simulink library "avalon_mm_alteradspbuilder2"  (Simulink 7.6)
settings: Solver=ode45  StartTime=0.0  StopTime=10.0  RelTol=1e-3
InitFcn:
  | %% DSPBuilder Start
  | alt_dspbuilder_update_model(bdroot)
  | %% DSPBuilder End
libraries: allblocks_alteradspbuilder2 x17
settings Model: Creator=swbuild  LastModifiedBy=swbuild

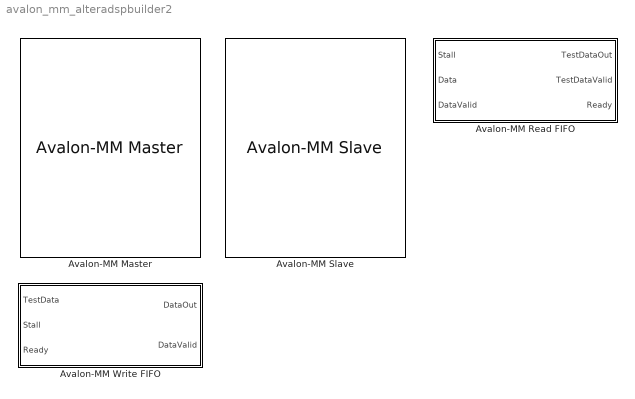
== system avalon_mm_alteradspbuilder2 ==
  Avalon-MM Master : allblocks_alteradspbuilder2/Avalon-MM Master  SystemSampleTime=-1  iofile=D:\avalon%5Fmm%5Falteradspbuilder2_Avalon-MM+Master_waitrequest.salt,D:\avalon%5Fmm%5Falteradspbuilder2_Avalon-MM+Master_address.capture,D:\avalon%5Fmm%5Falteradspbuilder2_Avalon-MM+Master_read.capture,D:\avalon%5Fmm%5Falteradspbuilder2_Avalon-MM+Master_readdata.salt,  SpecifyClock=off  addrWidth=2  addrType=Read  BusType=Signed Integer  bwl=8  bwr=0  byteEnable=off  flowCtrl=off  pipeline=off  flush=off  burst=off  maxBurst=4  irq=off  irq_mode=Prioritized  externalType=Inferred  PORTTYPE=Input
  Avalon-MM Read FIFO : Subsystem  mask(Avalon-MM Read FIFO AlteraBlockSet){sgn=Signed Integer, bwl=8, bwr=3, depth=11, burst=0}
      mask prompts: sgn "Data Type"; bwl "[number of bits].[]"; bwr "[].[number of bits]"; depth "FIFO Depth"; burst "Max Burst"
      mask help:
      | Avalon-MM Read FIFO
      |
      | Implements a FIFO with Avalon-MM connectivity. Accessed by other Avalon-MM peripherals to obtain datawhen connected in SOPC Builder.
      |
      | Inputs:
      | Stall - Connect to Simulink blocks.
      | 	Used to simulate stall conditions of the Avalon-MM bus.
      | Data - Connect to DSP Builder blocks.
      | 	Used to collect outgoing data from the user design.
      | DataValid - Connect to DSP Builder blocks.
      | 	Should be asserted whenever the signal on the Data port corresponds to real data.
      |
      | Outputs:
      | TestDataOut - Connect to Simulink blocks.
      | 	Corresponds to the data received over the Avalon-MM bus.
      | TestDataValid - Connect to Simulink blocks.
      | 	Asserted whenever TestDataOut corresponds to real data.
      | Ready	- Connect to DSP Builder blocks.
      | 	Used to indicate that the block is ready to receive data.
      mask init:
      | alt_dspbuilder_internal_AvalonFIFO_Init(gcb,1,1, bwl,bwr,depth,burst);
      settings: CopyFcn=set_param(gcbh,'LinkStatus','none');
      mask Help: helpview(fullfile(alt_dspbuilder_get_quartus_rootdir, 'dsp_builder', 'docs', 'AvalonReadFIFO.html'))
      mask StyleString: popup(Signed Integer|Signed Fractional|Unsigned Integer),edit,edit,edit,edit
      mask CallbackString: alt_dspbuilder_internal_AvalonFIFO_Init(gcb,1,0);||||
  Avalon-MM Slave : allblocks_alteradspbuilder2/Avalon-MM Slave  SystemSampleTime=-1  iofile=d:\SJ\nightly\13.1\162\w32\acds\quartus\dsp_builder\bin\mdllibrary\tb_avalon_mm_alteradspbuilder2\avalon%5Fmm%5Falteradspbuilder2_Avalon-MM+Slave_address.salt,d:\SJ\nightly\13.1\162\w32\acds\quartus\dsp_builder\bin\mdllibrary\tb_avalon_mm_alteradspbuilder2\avalon%5Fmm%5Falteradspbuilder2_Avalon-MM+Slave_write.salt,d:\SJ\nightly\13.1\162\w32\acds\quartus\dsp_builder\bin\mdllibrary\tb_avalon_mm_alteradspbuilder2\avalon%5Fmm%5Falteradspbuilder2_Avalon-MM+Slave_writedata.salt,d:\SJ\nightly\13.1\162\w32\acds\quartus\dsp_builder\bin\mdllibrary\tb_avalon_mm_alteradspbuilder2\avalon%5Fmm%5Falteradspbuilder2_Avalon-MM+Slave_byteenable.salt,  SpecifyClock=off  addrWidth=2  addrAlignment=Dynamic  addrType=Write  BusType=Unsigned Integer  bwl=16  bwr=0  byteEnable=on  flowCtrl=off  pipeline=off  waitStateFormat=Fixed  readWaitStateCycles=0  writeWaitStateCycles=0  readLatencyFormat=Fixed  readLatencyCycles=0  burst=off  maxBurst=4  irq=off  receiveBeginTransfer=off  useChipSelect=off  externalType=Inferred  PORTTYPE=Output
  Avalon-MM Write FIFO : Subsystem  mask(Avalon-MM Write FIFO AlteraBlockSet){sgn=Unsigned Integer, bwl=8, bwr=0, depth=16, burst=8}
      mask prompts: sgn "Data Type"; bwl "[number of bits].[]"; bwr "[].[number of bits]"; depth "FIFO Depth"; burst "Maximum Burst Size"
      mask help:
      | Avalon-MM Write FIFO
      |
      | Implements a FIFO with Avalon-MM connectivity. Used to receive data from other Avalon-MM peripheralswhen connected in SOPC Builder.
      |
      | Inputs:
      | TestData - Connect to Simulink blocks.
      | 	Used to provide simulation data to the Avalon-MM Write FIFO.
      | Stall - Connect to Simulink blocks.
      | 	Used to simulate stall conditions of the Avalon-MM bus.
      | Ready - Connect to DSP Builder blocks.
      | 	Used to indicate that the downstream hardware is ready for data.
      |
      | Outputs:
      | DataOut - Connect to DSP Builder blocks.
      | 	Corresponds to the oldest unsent data sample received on the TestData port.
      | DataValid - Connect to DSP Builder blocks.
      | 	Asserted whenever DataOut corresponds to real data.
      mask init:
      | alt_dspbuilder_internal_AvalonFIFO_Init(gcb,0,1, bwl,bwr,depth,burst);
      settings: CopyFcn=set_param(gcbh,'LinkStatus','none');
      mask Help: helpview(fullfile(alt_dspbuilder_get_quartus_rootdir, 'dsp_builder', 'docs', 'AvalonWriteFifo.html'))
      mask StyleString: popup(Signed Integer|Signed Fractional|Unsigned Integer),edit,edit,edit,edit
      mask CallbackString: alt_dspbuilder_internal_AvalonFIFO_Init(gcb,0,0);||||

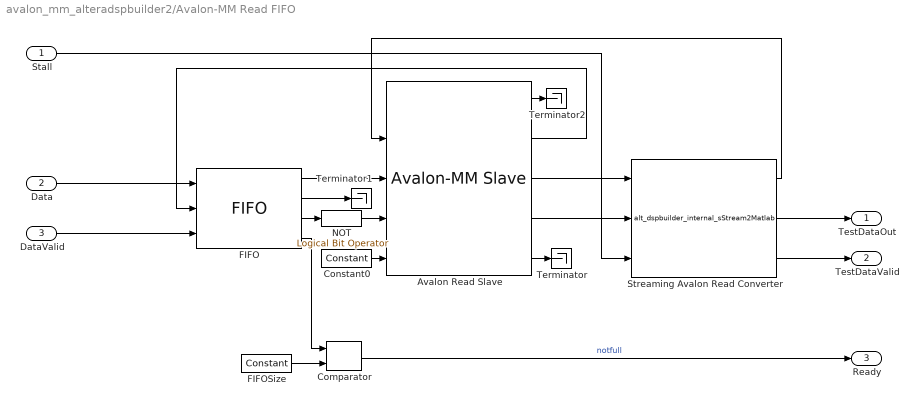
== system avalon_mm_alteradspbuilder2/Avalon-MM Read FIFO ==
  Stall : Inport
  Data : Inport  Port=2
  DataValid : Inport  Port=3
  Avalon Read Slave : allblocks_alteradspbuilder2/Avalon-MM Slave  SystemSampleTime=-1  iofile=d:\SJ\nightly\13.1\162\w32\acds\quartus\dsp_builder\bin\mdllibrary\tb_avalon_mm_alteradspbuilder2\avalon%5Fmm%5Falteradspbuilder2_Avalon-MM+Read+FIFO_Avalon+Read+Slave_address.salt,d:\SJ\nightly\13.1\162\w32\acds\quartus\dsp_builder\bin\mdllibrary\tb_avalon_mm_alteradspbuilder2\avalon%5Fmm%5Falteradspbuilder2_Avalon-MM+Read+FIFO_Avalon+Read+Slave_read.salt,d:\SJ\nightly\13.1\162\w32\acds\quartus\dsp_builder\bin\mdllibrary\tb_avalon_mm_alteradspbuilder2\avalon%5Fmm%5Falteradspbuilder2_Avalon-MM+Read+FIFO_Avalon+Read+Slave_readdata.capture,d:\SJ\nightly\13.1\162\w32\acds\quartus\dsp_builder\bin\mdllibrary\tb_avalon_mm_alteradspbuilder2\avalon%5Fmm%5Falteradspbuilder2_Avalon-MM+Read+FIFO_Avalon+Read+Slave_dataavailable.capture,d:\SJ\nightly\13.1\162\w32\acds\quartus\dsp_builder\bin\mdllibrary\tb_avalon_mm_alteradspbuilder2\avalon%5Fmm%5Falteradspbuilder2_Avalon-MM+Read+FIFO_Avalon+Read+Slave_endofpacket.capture,  SpecifyClock=off  clock=clock  addrWidth=2  addrAlignment=Dynamic  addrType=Read  BusType=Signed Integer  bwl=bwl  bwr=bwr  byteEnable=off  flowCtrl=on  pipeline=off  waitStateFormat=Fixed  readWaitStateCycles=0  writeWaitStateCycles=0  readLatencyFormat=Fixed  readLatencyCycles=0  burst=off  maxBurst=burst  irq=off  receiveBeginTransfer=off  useChipSelect=off  externalType=Inferred  PORTTYPE=Output
  Comparator : allblocks_alteradspbuilder2/Comparator  direction=a < b  pipeline_display=0  allowFloatingPointOverride=on  logOutputs=off  logFile=d:\SJ\nightly\13.1\162\w32\acds\quartus\dsp_builder\bin\mdllibrary\tb_avalon_mm_alteradspbuilder2\avalon%5Fmm%5Falteradspbuilder2_Avalon-MM+Read+FIFO_Comparator.fixedpointlog
  Constant0 : allblocks_alteradspbuilder2/Constant  mask_cst=0  BusType=Single Bit  bwl=1  bwr=0  roundMode=Truncate  satMode=Wrap  SpecifyClock=off  allowFloatingPointOverride=on  logOutputs=off  logFile=d:\SJ\nightly\13.1\162\w32\acds\quartus\dsp_builder\bin\mdllibrary\tb_avalon_mm_alteradspbuilder2\avalon%5Fmm%5Falteradspbuilder2_Avalon-MM+Read+FIFO_Constant0.fixedpointlog
  FIFO : allblocks_alteradspbuilder2/FIFO  numwords=depth  BusType=Signed Integer  bwl=bwl  bwr=bwr  ram_type=AUTO  use_sclr=off  use_les_only=off  showahead_mode=off  allowFloatingPointOverride=on  logOutputs=off  logFile=d:\SJ\nightly\13.1\162\w32\acds\quartus\dsp_builder\bin\mdllibrary\tb_avalon_mm_alteradspbuilder2\avalon%5Fmm%5Falteradspbuilder2_Avalon-MM+Read+FIFO_FIFO%3A%3Aq.fixedpointlog,d:\SJ\nightly\13.1\162\w32\acds\quartus\dsp_builder\bin\mdllibrary\tb_avalon_mm_alteradspbuilder2\avalon%5Fmm%5Falteradspbuilder2_Avalon-MM+Read+FIFO_FIFO%3A%3Afull.fixedpointlog,d:\SJ\nightly\13.1\162\w32\acds\quartus\dsp_builder\bin\mdllibrary\tb_avalon_mm_alteradspbuilder2\avalon%5Fmm%5Falteradspbuilder2_Avalon-MM+Read+FIFO_FIFO%3A%3Aempty.fixedpointlog,d:\SJ\nightly\13.1\162\w32\acds\quartus\dsp_builder\bin\mdllibrary\tb_avalon_mm_alteradspbuilder2\avalon%5Fmm%5Falteradspbuilder2_Avalon-MM+Read+FIFO_FIFO%3A%3Ausedw.fixedpointlog,
  FIFOSize : allblocks_alteradspbuilder2/Constant  mask_cst=depth - 2  BusType=Unsigned Integer  bwl=ceil(log2(depth -1))  bwr=0  roundMode=Truncate  satMode=Wrap  SpecifyClock=off  allowFloatingPointOverride=on  logOutputs=off  logFile=d:\SJ\nightly\13.1\162\w32\acds\quartus\dsp_builder\bin\mdllibrary\tb_avalon_mm_alteradspbuilder2\avalon%5Fmm%5Falteradspbuilder2_Avalon-MM+Read+FIFO_FIFOSize.fixedpointlog
  NOT : allblocks_alteradspbuilder2/Logical Bit Operator  LogicalOperator=NOT  user_inputs=2  pipeline_display=0
  Streaming Avalon Read Converter : S-Function  FunctionName=alt_dspbuilder_internal_sStream2Matlab  Parameters=-1  EnableBusSupport=off
      mask Display:
      | port_label('input', 1, 'ReadData');
      | port_label('input', 2, 'DataAvailable');
      | port_label('input', 3, 'Stall');
      | port_label('output', 1, 'Read');
      | port_label('output', 2, 'TestData');
      | port_label('output', 3, 'TestDataValid');
  Terminator : Terminator
  Terminator1 : Terminator
  Terminator2 : Terminator
  TestDataOut : Outport
  TestDataValid : Outport  Port=2
  Ready : Outport  Port=3
  wires:
  DataValid/1 -> FIFO/3
  FIFO/3 -> NOT/1
  NOT/1 -> Avalon Read Slave/4
  Data/1 -> FIFO/1
  FIFO/1 -> Avalon Read Slave/3
  Avalon Read Slave/2 -> FIFO/2
  Streaming Avalon Read Converter/2 -> TestDataOut/1
  Streaming Avalon Read Converter/3 -> TestDataValid/1
  Streaming Avalon Read Converter/1 -> Avalon Read Slave/2
  Avalon Read Slave/3 -> Streaming Avalon Read Converter/1
  Constant0/1 -> Avalon Read Slave/5
  FIFO/4 -> Comparator/1
  Comparator/1 -> Ready/1  "notfull"
  Stall/1 -> Streaming Avalon Read Converter/3
  Avalon Read Slave/4 -> Streaming Avalon Read Converter/2
  Avalon Read Slave/5 -> Terminator/1
  FIFOSize/1 -> Comparator/2
  FIFO/2 -> Terminator1/1
  Avalon Read Slave/1 -> Terminator2/1

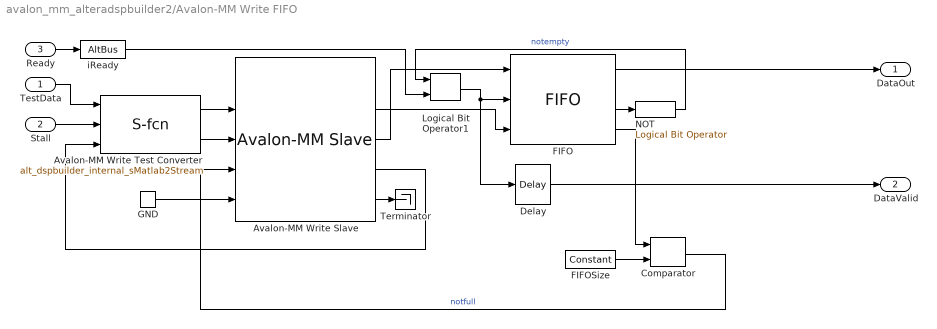
== system avalon_mm_alteradspbuilder2/Avalon-MM Write FIFO ==
  TestData : Inport
  Stall : Inport  Port=2
  Ready : Inport  Port=3
  Avalon-MM Write Slave : allblocks_alteradspbuilder2/Avalon-MM Slave  SystemSampleTime=-1  iofile=d:\SJ\nightly\13.1\162\w32\acds\quartus\dsp_builder\bin\mdllibrary\tb_avalon_mm_alteradspbuilder2\avalon%5Fmm%5Falteradspbuilder2_Avalon-MM+Write+FIFO_Avalon-MM+Write+Slave_address.salt,d:\SJ\nightly\13.1\162\w32\acds\quartus\dsp_builder\bin\mdllibrary\tb_avalon_mm_alteradspbuilder2\avalon%5Fmm%5Falteradspbuilder2_Avalon-MM+Write+FIFO_Avalon-MM+Write+Slave_write.salt,d:\SJ\nightly\13.1\162\w32\acds\quartus\dsp_builder\bin\mdllibrary\tb_avalon_mm_alteradspbuilder2\avalon%5Fmm%5Falteradspbuilder2_Avalon-MM+Write+FIFO_Avalon-MM+Write+Slave_writedata.salt,d:\SJ\nightly\13.1\162\w32\acds\quartus\dsp_builder\bin\mdllibrary\tb_avalon_mm_alteradspbuilder2\avalon%5Fmm%5Falteradspbuilder2_Avalon-MM+Write+FIFO_Avalon-MM+Write+Slave_readyfordata.capture,d:\SJ\nightly\13.1\162\w32\acds\quartus\dsp_builder\bin\mdllibrary\tb_avalon_mm_alteradspbuilder2\avalon%5Fmm%5Falteradspbuilder2_Avalon-MM+Write+FIFO_Avalon-MM+Write+Slave_endofpacket.capture,  SpecifyClock=off  clock=clock  addrWidth=2  addrAlignment=Dynamic  addrType=Write  BusType=Unsigned Integer  bwl=bwl  bwr=bwr  byteEnable=off  flowCtrl=on  pipeline=off  waitStateFormat=Fixed  readWaitStateCycles=0  writeWaitStateCycles=0  readLatencyFormat=Fixed  readLatencyCycles=0  burst=off  maxBurst=burst  irq=off  receiveBeginTransfer=off  useChipSelect=off  externalType=Inferred  PORTTYPE=Output
  Avalon-MM Write Test Converter : S-Function  FunctionName=alt_dspbuilder_internal_sMatlab2Stream  Parameters=-1 1000000  EnableBusSupport=off
      mask Display:
      | port_label('input', 1, 'TestData');
      | port_label('input', 2, 'Stall');
      | port_label('input', 3, 'Ready');
      | port_label('output', 1, 'Write');
      | port_label('output', 2, 'WriteData');
  Comparator : allblocks_alteradspbuilder2/Comparator  direction=a < b  pipeline_display=0  allowFloatingPointOverride=on  logOutputs=off  logFile=d:\SJ\nightly\13.1\162\w32\acds\quartus\dsp_builder\bin\mdllibrary\tb_avalon_mm_alteradspbuilder2\avalon%5Fmm%5Falteradspbuilder2_Avalon-MM+Write+FIFO_Comparator.fixedpointlog
  Delay : allblocks_alteradspbuilder2/Delay  pipeline=1  pipeline_display=1  ClockPhase=1  use_ena=off  use_sclr=off  allowFloatingPointOverride=on  logOutputs=off  logFile=d:\SJ\nightly\13.1\162\w32\acds\quartus\dsp_builder\bin\mdllibrary\tb_avalon_mm_alteradspbuilder2\avalon%5Fmm%5Falteradspbuilder2_Avalon-MM+Write+FIFO_Delay.fixedpointlog  use_init=off  reset_value=1
  FIFO : allblocks_alteradspbuilder2/FIFO  numwords=depth  BusType=Unsigned Integer  bwl=bwl  bwr=bwr  ram_type=AUTO  use_sclr=off  use_les_only=off  showahead_mode=off  allowFloatingPointOverride=on  logOutputs=off  logFile=d:\SJ\nightly\13.1\162\w32\acds\quartus\dsp_builder\bin\mdllibrary\tb_avalon_mm_alteradspbuilder2\avalon%5Fmm%5Falteradspbuilder2_Avalon-MM+Write+FIFO_FIFO%3A%3Aq.fixedpointlog,d:\SJ\nightly\13.1\162\w32\acds\quartus\dsp_builder\bin\mdllibrary\tb_avalon_mm_alteradspbuilder2\avalon%5Fmm%5Falteradspbuilder2_Avalon-MM+Write+FIFO_FIFO%3A%3Afull.fixedpointlog,d:\SJ\nightly\13.1\162\w32\acds\quartus\dsp_builder\bin\mdllibrary\tb_avalon_mm_alteradspbuilder2\avalon%5Fmm%5Falteradspbuilder2_Avalon-MM+Write+FIFO_FIFO%3A%3Aempty.fixedpointlog,d:\SJ\nightly\13.1\162\w32\acds\quartus\dsp_builder\bin\mdllibrary\tb_avalon_mm_alteradspbuilder2\avalon%5Fmm%5Falteradspbuilder2_Avalon-MM+Write+FIFO_FIFO%3A%3Ausedw.fixedpointlog,
  FIFOSize : allblocks_alteradspbuilder2/Constant  mask_cst=depth -2  BusType=Unsigned Integer  bwl=ceil(log2(depth-1))  bwr=0  roundMode=Truncate  satMode=Wrap  SpecifyClock=off  allowFloatingPointOverride=on  logOutputs=off  logFile=d:\SJ\nightly\13.1\162\w32\acds\quartus\dsp_builder\bin\mdllibrary\tb_avalon_mm_alteradspbuilder2\avalon%5Fmm%5Falteradspbuilder2_Avalon-MM+Write+FIFO_FIFOSize.fixedpointlog
  GND : allblocks_alteradspbuilder2/GND  SpecifyClock=off
  Logical Bit Operator1 : allblocks_alteradspbuilder2/Logical Bit Operator  LogicalOperator=AND  user_inputs=2  pipeline_display=0
  NOT : allblocks_alteradspbuilder2/Logical Bit Operator  LogicalOperator=NOT  user_inputs=2  pipeline_display=0
  Terminator : Terminator
  iReady : allblocks_alteradspbuilder2/AltBus  BusType=Single Bit  bwl=1  bwr=0  saturate=off  floatingPointInput=on  floatingPointOutput=on  logOutputs=off  logFile=D:\allblocks%5Falteradspbuilder2_Avalon-MM+Write+FIFO_iReady.fixedpointlog
  DataOut : Outport
  DataValid : Outport  Port=2
  wires:
  Ready/1 -> iReady/1
  Avalon-MM Write Slave/3 -> FIFO/1
  Avalon-MM Write Slave/2 -> FIFO/3
  FIFO/3 -> NOT/1
  FIFO/1 -> DataOut/1
  Avalon-MM Write Test Converter/1 -> Avalon-MM Write Slave/2
  Avalon-MM Write Slave/4 -> Avalon-MM Write Test Converter/3
  TestData/1 -> Avalon-MM Write Test Converter/1
  GND/1 -> Avalon-MM Write Slave/5
  NOT/1 -> Logical Bit Operator1/1  "notempty"
  iReady/1 -> Logical Bit Operator1/2
  Delay/1 -> DataValid/1
  Avalon-MM Write Test Converter/2 -> Avalon-MM Write Slave/3
  Stall/1 -> Avalon-MM Write Test Converter/2
  Avalon-MM Write Slave/5 -> Terminator/1
  Comparator/1 -> Avalon-MM Write Slave/4  "notfull"
  FIFOSize/1 -> Comparator/2
  FIFO/4 -> Comparator/1
  Logical Bit Operator1/1 -> FIFO/2, Delay/1
